simulink model "ex6continuo"  (R2015a)
settings: Solver=ode45  StartTime=0.0  StopTime=Tf  RelTol=1e-3
values from neighbouring files (symbols this model uses):
  C = K*tf([1 c], [1 p])    [C_zoh_approx_pade.m]    (also in ex6.m = (wn^2)*(s + c)/(s + 2*zeta*wn))
  G = 1/(s*(s+c))    [ex6.m]
settings Model: Creator=BPeixoto  LastModifiedBy=BPeixoto
settings DataIOCC: SaveFinalState=on  SaveCompleteFinalSimState=on  SaveFormat=StructureWithTime  SaveState=on

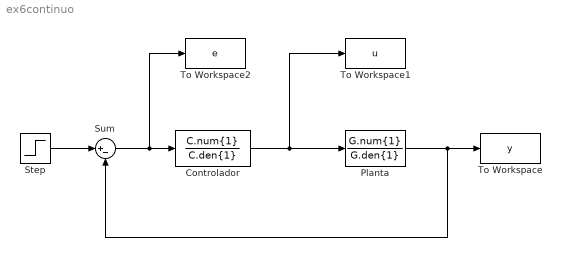
== system ex6continuo ==
  Controlador : TransferFcn  Numerator=C.num{1}  Denominator=C.den{1}
  Planta : TransferFcn  Numerator=G.num{1}  Denominator=G.den{1}
  Step : Step  Time=0  SampleTime=0
  Sum : Sum  Inputs=|+-
  To Workspace : ToWorkspace  VariableName=y  SaveFormat=Structure With Time  SampleTime=-1
  To Workspace1 : ToWorkspace  VariableName=u  SaveFormat=Structure With Time  SampleTime=-1
  To Workspace2 : ToWorkspace  VariableName=e  SaveFormat=Structure With Time  SampleTime=-1
  wires:
  Step/1 -> Sum/1
  Sum/1 -> To Workspace2/1, Controlador/1
  Planta/1 -> To Workspace/1, Sum/2
  Controlador/1 -> Planta/1, To Workspace1/1
